simulink model "q_sip_lqr"  (Simulink 7.8)
settings: Solver=ode4  StartTime=0.0  StopTime=inf  FixedStep=0.002  RelTol=1e-3
values from neighbouring files (symbols this model uses):
  A = [0 0 1 0 ... (first row only)    [SIP_ABCD_eqns.m]
  ALPHA_LIM_ENABLE = 1    [setup_ip02_sip.m]
  ALPHA_MAX = 20    [setup_ip02_sip.m]
  ALPHA_MIN = - ALPHA_MAX    (= -20)    [setup_ip02_sip.m]
  B = eta_g*Kg*eta_m*Kt/r_mp/Rm*B    [SIP_ABCD_eqns.m]
  C = eye(2,4)    [SIP_ABCD_eqns.m]    (also in d_ip02_sip_lqr.m = eye( 4 ))
  D = zeros(2,1)    [SIP_ABCD_eqns.m]    (also in d_ip02_sip_lqr.m = zeros( 4, 1 ))
  IC_ALPHA0 = IC_ALPHA0 / 180 * pi    (= 0)    [setup_ip02_sip.m]
  K_AMP = 1    [setup_ip02_sip.m]
  K_EC = Pr * N_pp / ( 4 * 1024 )    (= 2.27485440932e-05)    [config_ip02.m]
  K_EP = 2 * pi / ( 4 * 1024 )    (= 0.00153398078789)    [config_ip02.m]
  VMAX_AMP = 2.6 * IMAX_AMP    (= 4.16)    [config_ip02.m]
  VMAX_DAC = 10    [setup_ip02_sip.m]
  wcf = 2 * pi * 10.0    (= 62.8318530718)    [setup_ip02_sip.m]
  X_LIM_ENABLE = 1    [setup_ip02_sip.m]
  X_MAX = 0.3    [setup_ip02_sip.m]
  X_MIN = - X_MAX    (= -0.3)    [setup_ip02_sip.m]
  zetaf = 0.9    [setup_ip02_sip.m]
undefined symbols (not defined in the file or in its folder): HIL, K, qc_get_step_size
libraries: quarc_library x8, simulink_extras x3
settings Model: Creator=Mfotoohi  LastModifiedBy=pmartin  SimulationMode=external  ExtModeTrigDuration=5000
settings SolverCC: PositivePriorityOrder=on
settings OptimizationCC: BooleanDataType=off  InitFltsAndDblsToZero=on
settings DebuggingCC: SaveWithParameterizedLinksMsg=none  FcnCallInpInsideContextMsg=Use local settings  StrictBusMsg=Warning
settings RTWCC: SystemTargetFile=quarc_windows.tlc  TemplateMakefile=quarc_default_tmf  Description=Quarc Win32 Target  ProcessScript=quarc_windows_make_rtw_hook
settings STFCustomTargetCC: TargetFcnLib=ansi_tfl_tmw.mat  TargetPreCompLibLocation=C:\PROGRA~2\QUARC\lib\2011b\windows\release  SystemTargetFile=quarc_windows.tlc
settings GRTTargetCC: TargetFcnLib=ansi_tfl_tmw.mat  TargetPreCompLibLocation=C:\PROGRA~2\QUARC\lib\2011b\windows\release  ParMdlRefBuildCompliant=off  CompOptLevelCompliant=off  ConcurrentExecutionCompliant=off  MatFileLogging=off  ExtMode=on  ExtModeMexFile=quarc_comm

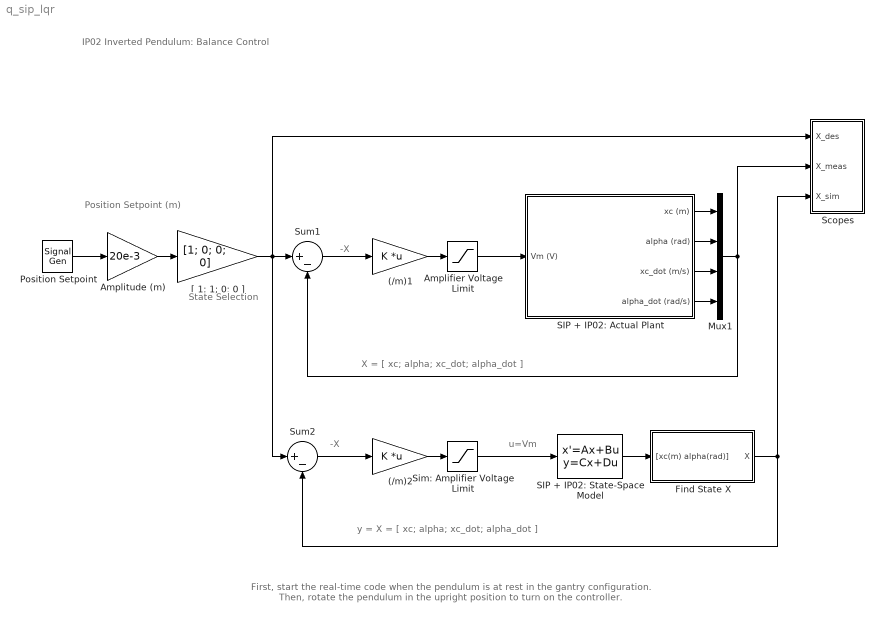
== system q_sip_lqr ==
  note: u=Vm
  note: X = [ xc; alpha; xc_dot; alpha_dot ]
  note: -X
  note: -X
  note: State Selection
  note: Position Setpoint (m)
  note: y = X = [ xc; alpha; xc_dot; alpha_dot ]
  note: First, start the real-time code when the pendulum is at rest in the gantry configuration.
      | Then, rotate the pendulum in the upright position to turn on the controller.
  note: IP02 Inverted Pendulum: Balance Control
  (/m)1 : Gain  Gain=K  Multiplication=Matrix(K*u)  SaturateOnIntegerOverflow=on  OutDataTypeStr=Inherit: Same as input  ParamDataTypeStr=Inherit: Same as input
  (/m)2 : Gain  Gain=K  Multiplication=Matrix(K*u)  SaturateOnIntegerOverflow=on  OutDataTypeStr=Inherit: Same as input  ParamDataTypeStr=Inherit: Same as input
  Amplifier Voltage Limit : Saturate  UpperLimit=VMAX_AMP  LowerLimit=- VMAX_AMP
  Amplitude (m) : Gain  Gain=20e-3  SaturateOnIntegerOverflow=on  OutDataTypeStr=Inherit: Same as input  ParamDataTypeStr=Inherit: Same as input
  Find State X : Subsystem
  Mux1 : Mux
  Position Setpoint : SignalGenerator  WaveForm=square  Frequency=0.1
  SIP + IP02: Actual Plant : Subsystem
  SIP + IP02: State-Space Model : StateSpace  A=A  B=B  C=C  D=D  X0=[ 0; IC_ALPHA0; 0; 0 ]
  Scopes : Subsystem
  Sim: Amplifier Voltage Limit : Saturate  UpperLimit=VMAX_AMP  LowerLimit=- VMAX_AMP
  Sum1 : Sum  Inputs=|+-  SaturateOnIntegerOverflow=on  InputSameDT=on  OutDataTypeStr=Inherit: Same as first input
  Sum2 : Sum  Inputs=|+-  SaturateOnIntegerOverflow=on  InputSameDT=on  OutDataTypeStr=Inherit: Same as first input
  "[ 1; 1; 0; 0 ]" : Gain  Gain=[1; 0; 0; 0]  SaturateOnIntegerOverflow=on  OutDataTypeStr=Inherit: Same as input  ParamDataTypeStr=Inherit: Same as input
  wires:
  SIP + IP02: Actual Plant/1(xc (m)) -> Mux1/1
  SIP + IP02: Actual Plant/2(alpha (rad)) -> Mux1/2
  SIP + IP02: Actual Plant/4(alpha_dot (rad/s)) -> Mux1/4
  (/m)2/1 -> Sim: Amplifier Voltage Limit/1
  Sum2/1 -> (/m)2/1
  "[ 1; 1; 0; 0 ]"/1 -> Sum1/1, Scopes/1(X_des), Sum2/1
  Mux1/1 -> Scopes/2(X_meas), Sum1/2
  SIP + IP02: Actual Plant/3(xc_dot (m/s)) -> Mux1/3
  Position Setpoint/1 -> Amplitude (m)/1
  Amplitude (m)/1 -> "[ 1; 1; 0; 0 ]"/1
  Sum1/1 -> (/m)1/1
  (/m)1/1 -> Amplifier Voltage Limit/1
  Amplifier Voltage Limit/1 -> SIP + IP02: Actual Plant/1(Vm (V))
  Sim: Amplifier Voltage Limit/1 -> SIP + IP02: State-Space Model/1
  SIP + IP02: State-Space Model/1 -> Find State X/1("[xc(m) alpha(rad)]")
  Find State X/1(X) -> Sum2/2, Scopes/3(X_sim)

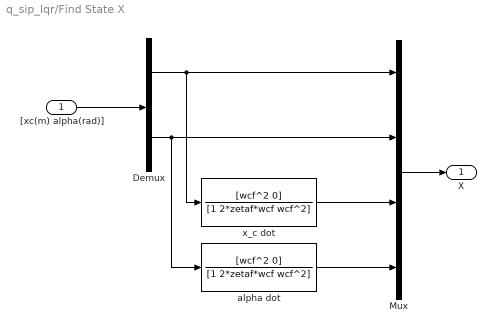
== system q_sip_lqr/Find State X ==
  "[xc(m) alpha(rad)]" : Inport
  Demux : Demux  Outputs=2
  Mux : Mux
  alpha dot : TransferFcn  Numerator=[wcf^2 0]  Denominator=[1 2*zetaf*wcf wcf^2]
  x_c dot : TransferFcn  Numerator=[wcf^2 0]  Denominator=[1 2*zetaf*wcf wcf^2]
  X : Outport
  wires:
  Mux/1 -> X/1
  x_c dot/1 -> Mux/3
  alpha dot/1 -> Mux/4
  "[xc(m) alpha(rad)]"/1 -> Demux/1
  Demux/1 -> Mux/1, x_c dot/1
  Demux/2 -> Mux/2, alpha dot/1

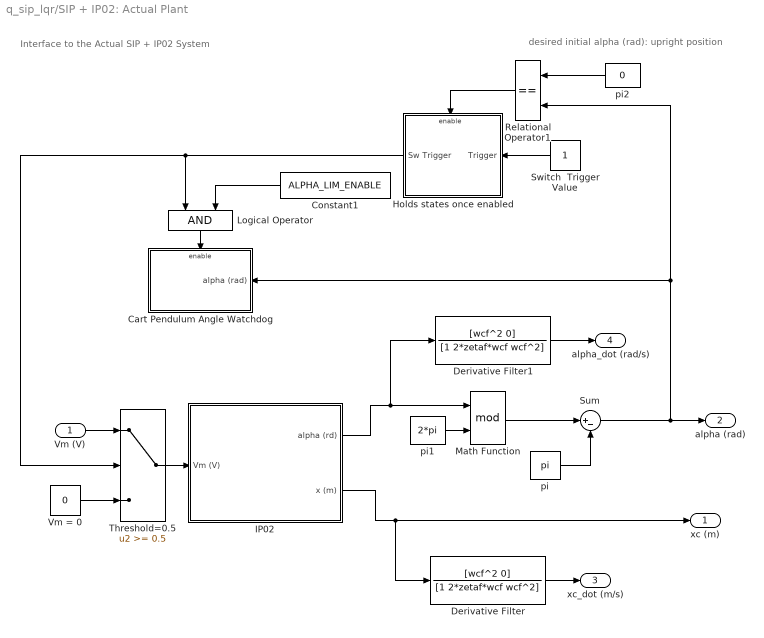
== system q_sip_lqr/SIP + IP02: Actual Plant ==
  note: Interface to the Actual
      | SIP + IP02 System
  note: desired initial alpha (rad):
      | upright position
  Vm (V) : Inport
  Cart Pendulum Angle Watchdog : Subsystem  TreatAsAtomicUnit=on
  Constant1 : Constant  Value=ALPHA_LIM_ENABLE  OutDataTypeStr=double
  Derivative Filter : TransferFcn  Numerator=[wcf^2 0]  Denominator=[1 2*zetaf*wcf wcf^2]
  Derivative Filter1 : TransferFcn  Numerator=[wcf^2 0]  Denominator=[1 2*zetaf*wcf wcf^2]
  Holds states once enabled : Subsystem  TreatAsAtomicUnit=on
  "IP02 " : Subsystem
  Logical Operator : Logic
  Math Function : Math  Operator=mod  SaturateOnIntegerOverflow=on
  Relational Operator1 : RelationalOperator  Operator===  InputSameDT=on
  Sum : Sum  Inputs=|+-  SaturateOnIntegerOverflow=on  InputSameDT=on  OutDataTypeStr=Inherit: Same as first input
  Switch  Trigger Value : Constant
  Threshold=0.5 : Switch  Threshold=0.5  SaturateOnIntegerOverflow=on  InputSameDT=on
  Vm = 0 : Constant  Value=0
  pi : Constant  Value=pi
  pi1 : Constant  Value=2*pi
  pi2 : Constant  Value=0
  xc (m) : Outport  InitialOutput=0
  alpha (rad) : Outport  Port=2  InitialOutput=0
  xc_dot (m/s) : Outport  Port=3  InitialOutput=0
  alpha_dot (rad/s) : Outport  Port=4  InitialOutput=0
  wires:
  "IP02 "/2(x (m)) -> xc (m)/1, Derivative Filter/1
  Derivative Filter1/1 -> alpha_dot (rad/s)/1
  "IP02 "/1(alpha (rd)) -> Derivative Filter1/1, Math Function/1
  Derivative Filter/1 -> xc_dot (m/s)/1
  pi1/1 -> Math Function/2
  pi2/1 -> Relational Operator1/1
  Switch  Trigger Value/1 -> Holds states once enabled/1(Trigger)
  Relational Operator1/1 -> Holds states once enabled/Enable
  Threshold=0.5/1 -> "IP02 "/1(Vm (V))
  Holds states once enabled/1(Sw Trigger) -> Threshold=0.5/2, Logical Operator/1
  Vm = 0/1 -> Threshold=0.5/3
  pi/1 -> Sum/2
  Sum/1 -> alpha (rad)/1, Relational Operator1/2, Cart Pendulum Angle Watchdog/1(alpha (rad))
  Math Function/1 -> Sum/1
  Logical Operator/1 -> Cart Pendulum Angle Watchdog/Enable
  Constant1/1 -> Logical Operator/2
  Vm (V)/1 -> Threshold=0.5/1

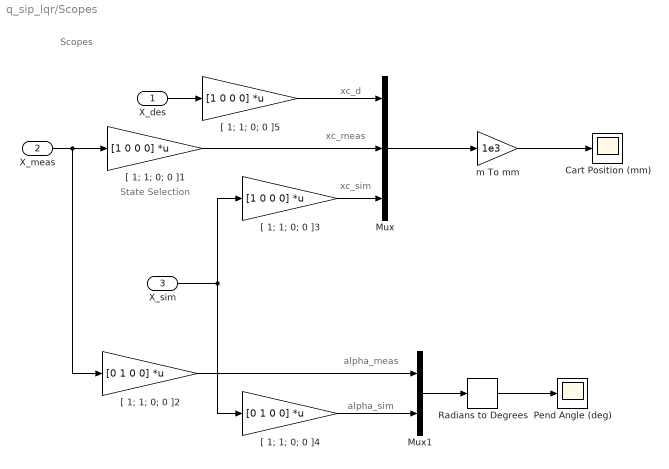
== system q_sip_lqr/Scopes ==
  note: xc_meas
  note: State Selection
  note: alpha_meas
  note: alpha_sim
  note: xc_sim
  note: xc_d
  note: Scopes
  X_des : Inport
  X_meas : Inport  Port=2
  X_sim : Inport  Port=3
  Cart Position (mm) : Scope
      settings: TickLabels=on  TimeRange=10  YMin=-80  YMax=70  SaveName=data_xc  DataFormat=Array
  Mux : Mux  Inputs=3
  Mux1 : Mux  Inputs=2
  Pend Angle (deg) : Scope
      settings: TickLabels=on  TimeRange=10  YMin=-180  YMax=10  SaveName=data_alpha  DataFormat=Array
  Radians to Degrees : simulink_extras/Transformations/Radians to Degrees
  "[ 1; 1; 0; 0 ]1" : Gain  Gain=[1 0 0 0]  Multiplication=Matrix(K*u)  SaturateOnIntegerOverflow=on  OutDataTypeStr=Inherit: Same as input  ParamDataTypeStr=Inherit: Same as input
  "[ 1; 1; 0; 0 ]2" : Gain  Gain=[0 1 0 0]  Multiplication=Matrix(K*u)  SaturateOnIntegerOverflow=on  OutDataTypeStr=Inherit: Same as input  ParamDataTypeStr=Inherit: Same as input
  "[ 1; 1; 0; 0 ]3" : Gain  Gain=[1 0 0 0]  Multiplication=Matrix(K*u)  SaturateOnIntegerOverflow=on  OutDataTypeStr=Inherit: Same as input  ParamDataTypeStr=Inherit: Same as input
  "[ 1; 1; 0; 0 ]4" : Gain  Gain=[0 1 0 0]  Multiplication=Matrix(K*u)  SaturateOnIntegerOverflow=on  OutDataTypeStr=Inherit: Same as input  ParamDataTypeStr=Inherit: Same as input
  "[ 1; 1; 0; 0 ]5" : Gain  Gain=[1 0 0 0]  Multiplication=Matrix(K*u)  SaturateOnIntegerOverflow=on  OutDataTypeStr=Inherit: Same as input  ParamDataTypeStr=Inherit: Same as input
  m To mm : Gain  Gain=1e3  SaturateOnIntegerOverflow=on  OutDataTypeStr=Inherit: Same as input  ParamDataTypeStr=Inherit: Same as input
  wires:
  Mux/1 -> m To mm/1
  m To mm/1 -> Cart Position (mm)/1
  "[ 1; 1; 0; 0 ]1"/1 -> Mux/2
  X_des/1 -> "[ 1; 1; 0; 0 ]5"/1
  X_meas/1 -> "[ 1; 1; 0; 0 ]1"/1, "[ 1; 1; 0; 0 ]2"/1
  Mux1/1 -> Radians to Degrees/1
  Radians to Degrees/1 -> Pend Angle (deg)/1
  X_sim/1 -> "[ 1; 1; 0; 0 ]3"/1, "[ 1; 1; 0; 0 ]4"/1
  "[ 1; 1; 0; 0 ]3"/1 -> Mux/3
  "[ 1; 1; 0; 0 ]5"/1 -> Mux/1
  "[ 1; 1; 0; 0 ]2"/1 -> Mux1/1
  "[ 1; 1; 0; 0 ]4"/1 -> Mux1/2

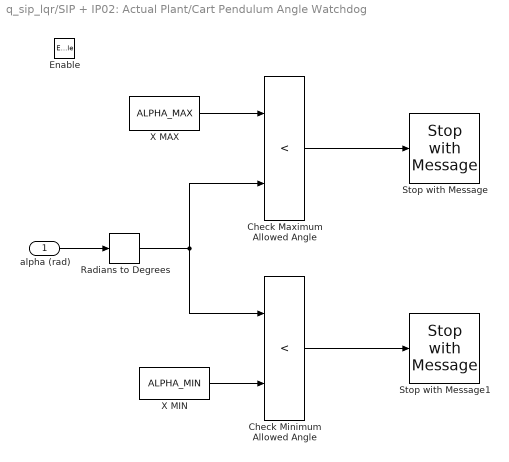
== system q_sip_lqr/SIP + IP02: Actual Plant/Cart Pendulum Angle Watchdog ==
  alpha (rad) : Inport
  Enable : EnablePort
  Check Maximum Allowed Angle : RelationalOperator  Operator=<  InputSameDT=on
  Check Minimum Allowed Angle : RelationalOperator  Operator=<  InputSameDT=on
  Radians to Degrees : simulink_extras/Transformations/Radians to Degrees
  Stop with Message : quarc_library/Sinks/Error Handling/Stop with Message  message_type=Fixed error message  message_icon=Error  message=Maximum Angle Reached.
  Stop with Message1 : quarc_library/Sinks/Error Handling/Stop with Message  message_type=Fixed error message  message_icon=Error  message=Minimum Angle Reached.
  X MAX : Constant  Value=ALPHA_MAX
  X MIN : Constant  Value=ALPHA_MIN
  wires:
  X MAX/1 -> Check Maximum Allowed Angle/1
  Check Minimum Allowed Angle/1 -> Stop with Message1/1
  X MIN/1 -> Check Minimum Allowed Angle/2
  alpha (rad)/1 -> Radians to Degrees/1
  Check Maximum Allowed Angle/1 -> Stop with Message/1
  Radians to Degrees/1 -> Check Maximum Allowed Angle/2, Check Minimum Allowed Angle/1

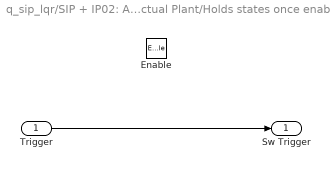
== system q_sip_lqr/SIP + IP02: Actual Plant/Holds states once enabled ==
  Trigger : Inport  OutDataTypeStr=double
  Enable : EnablePort
  Sw Trigger : Outport  OutDataTypeStr=double  InitialOutput=[0]
  wires:
  Trigger/1 -> Sw Trigger/1

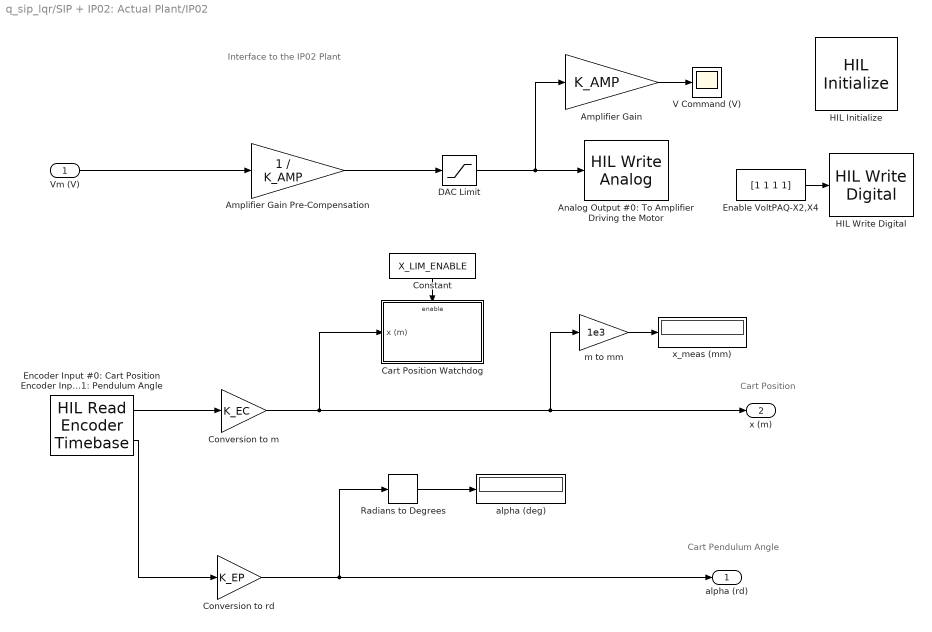
== system q_sip_lqr/SIP + IP02: Actual Plant/IP02  ==
  note: Cart Pendulum Angle
  note: Cart Position
  note: Interface to the IP02 Plant
  Vm (V) : Inport
  Amplifier Gain : Gain  Gain=K_AMP  SaturateOnIntegerOverflow=on  OutDataTypeStr=Inherit: Same as input  ParamDataTypeStr=Inherit: Same as input
  Amplifier Gain Pre-Compensation : Gain  Gain=1 / K_AMP  SaturateOnIntegerOverflow=on  OutDataTypeStr=Inherit: Same as input  ParamDataTypeStr=Inherit: Same as input
  Analog Output #0: To Amplifier Driving the Motor : quarc_library/Data Acquisition/Generic/Immediate I//O/HIL Write Analog  Tag=unassigned  object_name=HIL-1  channels=0  sample_time=-1  active=on  vector_input=on
  Cart Position Watchdog : Subsystem  TreatAsAtomicUnit=on
  Constant : Constant  Value=X_LIM_ENABLE
  Conversion to m : Gain  Gain=K_EC  SaturateOnIntegerOverflow=on  OutDataTypeStr=Inherit: Same as input  ParamDataTypeStr=Inherit: Same as input
  Conversion to rd : Gain  Gain=K_EP  SaturateOnIntegerOverflow=on  OutDataTypeStr=Inherit: Same as input  ParamDataTypeStr=Inherit: Same as input
  DAC Limit : Saturate  UpperLimit=VMAX_DAC  LowerLimit=- VMAX_DAC
  Enable VoltPAQ-X2,X4 : Constant  Value=[1 1 1 1]
  Encoder Input #0: Cart Position Encoder Input #1: Pendulum Angle : quarc_library/Data Acquisition/Generic/Timebases/HIL Read Encoder Timebase  Tag=unassigned  object_name=HIL-1  clock=0  channels=[0 1]  samples_in_buffer=max(ceil(1/qc_get_step_size), 1)  active=on  vector_output=off  data_type_mode=Inherit via back propagation  data_type=double
  HIL Initialize : quarc_library/Data Acquisition/Generic/Configuration/HIL Initialize  object_name=HIL-1  board_type=q2_usb  board_number=0  board_options=d0=digital;d1=digital;led=auto;update_rate=normal  exclusive=off  active=off  hardware_clocks=[0:2]  clock_modes=[]  initial_clock_frequencies=[]  set_clock_params_at_start=off  set_clock_params_at_switch_in=off  set_clock_frequencies_at_start=off  set_clock_frequencies_at_switch_in=off  analog_input_channels=[0:1]  analog_input_maximums=10  analog_input_minimums=-10  set_analog_input_params_at_start=on  set_analog_input_params_at_switch_in=off  analog_output_channels=[0:1]  analog_output_maximums=10  analog_output_minimums=-10  initial_analog_outputs=[0]  final_analog_outputs=[0]  watchdog_analog_outputs=0  set_analog_output_params_at_start=on  set_analog_output_params_at_switch_in=off  set_analog_outputs_at_start=on  set_analog_outputs_at_switch_in=off  set_analog_outputs_at_terminate=on  set_analog_outputs_at_switch_out=off  set_analog_outputs_on_watchdog=off  digital_input_channels=[]  digital_output_channels=[0:7]  digital_output_configuration=[]  initial_digital_outputs=[0]  final_digital_outputs=[0]  watchdog_digital_outputs=[0]  set_digital_output_params_at_start=off  set_digital_output_params_at_switch_in=off  set_digital_outputs_at_start=on  set_digital_outputs_at_switch_in=off  set_digital_outputs_at_terminate=on  set_digital_outputs_at_switch_out=off  set_digital_outputs_on_watchdog=off  encoder_channels=[0:1]  quadrature=[4]  encoder_filter_frequency=[]  initial_encoder_counts=[0]  set_encoder_params_at_start=on  set_encoder_params_at_switch_in=off  set_encoder_counts_at_start=on  set_encoder_counts_at_switch_in=off  pwm_channels=[]  pwm_modes=[0]  pwm_frequency=1/0.020  pwm_configuration=[]  pwm_alignment=[]  pwm_polarity=[]  pwm_leading_deadband=[]  pwm_trailing_deadband=[]  initial_pwm_outputs=[0]  final_pwm_outputs=[0]  watchdog_pwm_outputs=[0]  set_pwm_params_at_start=on  set_pwm_params_at_switch_in=off  set_pwm_outputs_at_start=on  set_pwm_outputs_at_switch_in=off  set_pwm_outputs_at_terminate=on  set_pwm_outputs_at_switch_out=off  set_pwm_outputs_on_watchdog=off  other_output_channels=[]  initial_other_outputs=[]  final_other_outputs=[]  watchdog_other_outputs=[]  set_other_outputs_at_start=off  set_other_outputs_at_switch_in=off  set_other_outputs_at_terminate=off  set_other_outputs_at_switch_out=off  set_other_outputs_on_watchdog=off
  HIL Write Digital : quarc_library/Data Acquisition/Generic/Immediate I//O/HIL Write Digital  object_name=HIL-1  channels=[0:3]  sample_time=-1  active=off  vector_input=on
  Radians to Degrees : simulink_extras/Transformations/Radians to Degrees
  V Command (V) : Scope
      settings: TickLabels=on  TimeRange=10  YMin=-6  YMax=6  SaveName=data_Vm  DataFormat=Array
  alpha (deg) : Display
      settings: Decimation=100
  m to mm : Gain  Gain=1e3  SaturateOnIntegerOverflow=on  OutDataTypeStr=Inherit: Same as input  ParamDataTypeStr=Inherit: Same as input
  x_meas (mm) : Display
      settings: Decimation=100
  alpha (rd) : Outport  InitialOutput=0
  x (m) : Outport  Port=2  InitialOutput=0
  wires:
  Encoder Input #0: Cart Position Encoder Input #1: Pendulum Angle/1 -> Conversion to m/1
  Conversion to m/1 -> Cart Position Watchdog/1(x (m)), x (m)/1, m to mm/1
  Amplifier Gain Pre-Compensation/1 -> DAC Limit/1
  m to mm/1 -> x_meas (mm)/1
  Encoder Input #0: Cart Position Encoder Input #1: Pendulum Angle/2 -> Conversion to rd/1
  Radians to Degrees/1 -> alpha (deg)/1
  Conversion to rd/1 -> Radians to Degrees/1, alpha (rd)/1
  Constant/1 -> Cart Position Watchdog/Enable
  DAC Limit/1 -> Analog Output #0: To Amplifier Driving the Motor/1, Amplifier Gain/1
  Vm (V)/1 -> Amplifier Gain Pre-Compensation/1
  Amplifier Gain/1 -> V Command (V)/1
  Enable VoltPAQ-X2,X4/1 -> HIL Write Digital/1

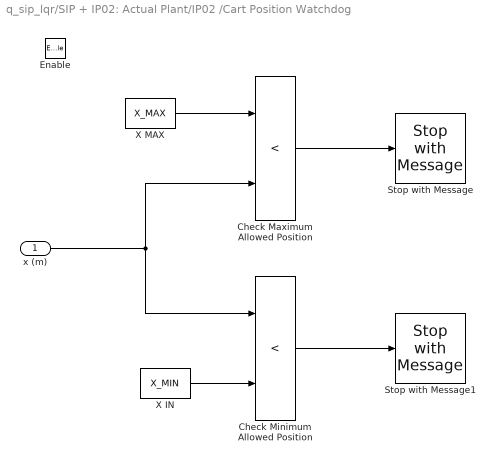
== system q_sip_lqr/SIP + IP02: Actual Plant/IP02 /Cart Position Watchdog ==
  x (m) : Inport
  Enable : EnablePort
  Check Maximum Allowed Position : RelationalOperator  Operator=<  InputSameDT=on
  Check Minimum Allowed Position : RelationalOperator  Operator=<  InputSameDT=on
  Stop with Message : quarc_library/Sinks/Error Handling/Stop with Message  message_type=Fixed error message  message_icon=Error  message=Maximum Limit Reached.
  Stop with Message1 : quarc_library/Sinks/Error Handling/Stop with Message  message_type=Fixed error message  message_icon=Error  message=Minimum Limit Reached.
  X IN : Constant  Value=X_MIN
  X MAX : Constant  Value=X_MAX
  wires:
  Check Maximum Allowed Position/1 -> Stop with Message/1
  x (m)/1 -> Check Minimum Allowed Position/1, Check Maximum Allowed Position/2
  X IN/1 -> Check Minimum Allowed Position/2
  Check Minimum Allowed Position/1 -> Stop with Message1/1
  X MAX/1 -> Check Maximum Allowed Position/1
